simulink model "dspstsa"  (Simulink 6.0)
settings: Solver=FixedStepDiscrete  StartTime=0.0  StopTime=4.99  FixedStep=1/22050  RelTol=1e-3
undefined symbols (not defined in the file or in its folder): magnitude
libraries: dspxfrm3 x2, simulink x1, dspsrcs4 x1, dspwin32 x1
settings Model: Creator=mani  LastModifiedBy=schim  ExtModeTrigMode=oneshot  ExtModeArmWhenConnect=off  ExtModeAutoUpdateStatusClock=off  ProdHWDeviceType=Specified
settings DataIOCC: LimitDataPoints=off  SaveOutput=off  SaveTime=off  SignalLoggingName=sigsOut
settings OptimizationCC: InlineParams=on
settings DebuggingCC: CheckExecutionContextPreStartOutputMsg=on  CheckExecutionContextRuntimeOutputMsg=on  SolverPrmCheckMsg=none
settings HardwareCC: ProdBitPerShort=32  ProdBitPerInt=16  ProdHWDeviceType=Specified  TargetUnknown=on
settings SFSimCC: SFSimApplyToAllLibs=on  SFSimBuildMode=Incremental

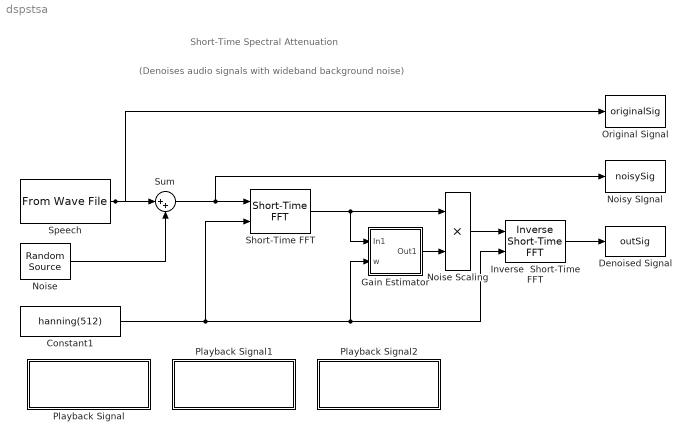
== system dspstsa ==
  note: Short-Time Spectral Attenuation
  note: (Denoises audio signals with wideband background noise)
  Constant1 : Constant  Value=hanning(512)
  Denoised Signal : ToWorkspace  VariableName=outSig  SampleTime=-1  SaveFormat=Array
  Gain Estimator : Subsystem  PropExecContextAcrossSSBoundary=on  mask(Estimate Gain for Noise Suppression){noiseStd=0.05, decimat=16, alpha=15}
      mask prompts: noiseStd "Noise Standard Deviation:"; decimat "Decimation:"; alpha "Weighting (alpha):"
      mask Display: disp(sprintf('Gain\n Estimator'))
  Inverse  Short-Time FFT : dspxfrm3/Inverse  Short-Time FFT  OvLap=512-16  OutFrameSize=512  InConjSymm=on  DoAssert=off  W=512  Tol=1e-4
  Noise : dspsrcs4/Random Source  SrcType=Gaussian  NormMethod=Ziggurat  CltLength=12  Min=0  Max=1  Mean=0  Var=(0.05)^2  RepMode=Not repeatable  rawSeed=1  Inherit=off  SampMode=Discrete  SampTime=1/22050  SampFrame=512  DataType=Double  OutComplex=Real
  Noise Scaling : Product  InputSameDT=on
  Noisy SIgnal : ToWorkspace  VariableName=noisySig  SampleTime=-1  SaveFormat=Array
  Original Signal : ToWorkspace  VariableName=originalSig  SampleTime=-1  SaveFormat=Array
  Playback Signal : Subsystem  PropExecContextAcrossSSBoundary=on
      settings: OpenFcn=|
      | [y,Fs]=wavread('speech_dft.wav');
      | p=audioplayer(y,Fs);
      | play(p)
      mask Type: Original Signal
      mask Display: disp('Playback\nOriginal Signal')
  Playback Signal1 : Subsystem  PropExecContextAcrossSSBoundary=on
      settings: OpenFcn=|
      | if exist('noisySig','var'),
      |    pNois=audioplayer(noisySig,22050);
      |   play(pNois)
      | else
      |    errordlg('Run model before playing.', ...
      |                'Signal Processing Blockset Demo Error');
      | end
      mask Type: Original Signal
      mask Display: disp('Playback\nNoisy Signal')
  Playback Signal2 : Subsystem  PropExecContextAcrossSSBoundary=on
      settings: OpenFcn=|
      | if exist('outSig','var'),
      |    pDeNois=audioplayer(outSig,22050);
      |    play(pDeNois)
      | else
      |    errordlg('Run model before playing.', ...
      |                'Signal Processing Blockset Demo Error');
      | end
      mask Type: Original Signal
      mask Display: disp('Playback\nDenoised Signal')
  Short-Time FFT : dspxfrm3/Short-Time FFT  W=512  OvLap=512-16  M=1024
  Speech : dspwin32/From Wave File  FileName=speech_dft.wav  SamplesPerFrame=512  MinBufSize=512  dType=double  bLoop=off  timesToPlay=1  restartMode=immediately after last sample  firstSampleOutput=off  lastSampleOutput=off
  Sum : Sum  Inputs=|++  SaturateOnIntegerOverflow=on  InputSameDT=on
  wires:
  Speech/1 -> Sum/1, Original Signal/1
  Noise/1 -> Sum/2
  Sum/1 -> Noisy SIgnal/1, Short-Time FFT/1
  Constant1/1 -> Gain Estimator/2(w), Inverse  Short-Time FFT/2, Short-Time FFT/2
  Inverse  Short-Time FFT/1 -> Denoised Signal/1
  Noise Scaling/1 -> Inverse  Short-Time FFT/1
  Short-Time FFT/1 -> Noise Scaling/1, Gain Estimator/1(In1)
  Gain Estimator/1(Out1) -> Noise Scaling/2

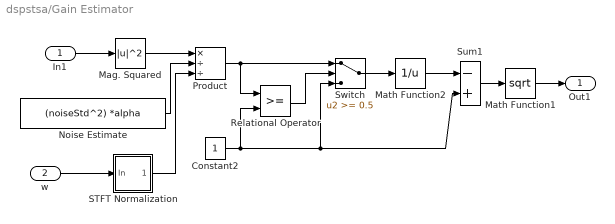
== system dspstsa/Gain Estimator ==
  In1 : Inport  LatchInput=off
  w : Inport  Port=2  LatchInput=off
  Constant2 : Constant
  Mag. Squared : Math  Operator=magnitude^2  SaturateOnIntegerOverflow=on
  Math Function1 : Math  Operator=sqrt  SaturateOnIntegerOverflow=on
  Math Function2 : Math  Operator=reciprocal  SaturateOnIntegerOverflow=on
  Noise Estimate : Constant  Value=(noiseStd^2) *alpha
  Product : Product  Inputs=*//  SaturateOnIntegerOverflow=on  InputSameDT=on
  Relational Operator : RelationalOperator  InputSameDT=on
  STFT Normalization : Subsystem  PropExecContextAcrossSSBoundary=on
  Sum1 : Sum  Inputs=-+  SaturateOnIntegerOverflow=on  InputSameDT=on
  Switch : Switch  Threshold=0.5  SaturateOnIntegerOverflow=on  InputSameDT=on
  Out1 : Outport
  wires:
  Mag. Squared/1 -> Product/1
  In1/1 -> Mag. Squared/1
  Noise Estimate/1 -> Product/2
  Constant2/1 -> Relational Operator/2, Switch/3, Sum1/2
  Switch/1 -> Math Function2/1
  Relational Operator/1 -> Switch/2
  Product/1 -> Relational Operator/1, Switch/1
  Math Function2/1 -> Sum1/1
  Math Function1/1 -> Out1/1
  Sum1/1 -> Math Function1/1
  w/1 -> STFT Normalization/1(In)
  STFT Normalization/1(Out) -> Product/3

== system dspstsa/Playback Signal ==

== system dspstsa/Playback Signal1 ==

== system dspstsa/Playback Signal2 ==

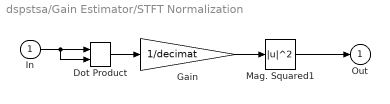
== system dspstsa/Gain Estimator/STFT Normalization ==
  In : Inport  LatchInput=off
  Dot Product : simulink/Math Operations/Dot Product  OutDataType=sfix(16)  OutScaling=2^-10  DoSatur=off
  Gain : Gain  Gain=1/decimat  SaturateOnIntegerOverflow=on
  Mag. Squared1 : Math  Operator=magnitude^2  SaturateOnIntegerOverflow=on
  Out : Outport
  wires:
  Dot Product/1 -> Gain/1
  In/1 -> Dot Product/1, Dot Product/2
  Gain/1 -> Mag. Squared1/1
  Mag. Squared1/1 -> Out/1
